simulink model "PS3"  (Simulink 7.3)
settings: Solver=ode5  StartTime=0.0  StopTime=inf  FixedStep=0.1  RelTol=1e-3
libraries: simulink x18, dspinverses x1
settings Model: Creator=Dinh  LastModifiedBy=mcl  BufferReuse=off
settings DataIOCC: LimitDataPoints=off  SaveOutput=off  SaveTime=off
settings OptimizationCC: BlockReduction=off  BooleanDataType=off  ConditionallyExecuteInputs=off  OptimizeBlockIOStorage=off  BufferReuse=off  ExpressionFolding=off  LocalBlockOutputs=off  SimCompilerOptimization=On
settings SFSimCC: SimBuildMode=sf_nonincremental_build
settings RTWCC: SystemTargetFile=nidll.tlc  TemplateMakefile=nidll_vc.tmf  Description=NI Real-Time Target for Release 2007b or later  ProcessScript=nidll_make_rtw_hook
settings STFCustomTargetCC: MatFileLogging=on  SystemTargetFile=nidll.tlc

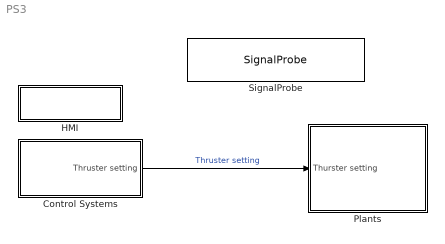
== system PS3 ==
  Control Systems : Subsystem
  HMI : Subsystem
  Plants : Subsystem
  SignalProbe : S-Function  Description=Use this block with SIT.  FunctionName=SignalProbe  Parameters=1  EnableBusSupport=off
      settings: PreSaveFcn=NISIT_ModelVars;
      mask Description: The LabVIEW Simulation Interface Toolkit uses the SignalProbe block to probe the signals in the model. The SignalProbe block must be on the top level of the model hierarchy. You can have only one SignalProbe block per model file. Do not rename the SignalProbe block. Do not change the name of another model block to SignalProbe.
  wires:
  Control Systems/1(Thruster setting) -> Plants/1(Thurster setting)  "Thruster setting"

== system PS3/Control Systems ==
  note: 0 - PS3 u input control
      | 1 - PS3 tau input control
  Control Mode : Constant  Value=0
  PS3 input : Subsystem
  PS3 tau input control : Subsystem
      settings: MinAlgLoopOccurrences=on
  PS3 u input control : Subsystem
      settings: MinAlgLoopOccurrences=on
  Saturation : Saturate  UpperLimit=1.0  LowerLimit=-1.0
  Thruster setting Switch : MultiPortSwitch  Inputs=2  zeroidx=on
  Thruster setting : Outport  PortDimensions=7
  wires:
  Thruster setting Switch/1 -> Saturation/1
  Saturation/1 -> Thruster setting/1
  PS3 input/1(DuelShock 3 signals) -> PS3 u input control/1(PS3 Signals), PS3 tau input control/1(PS3 Signals)
  PS3 input/2(PS3 BT Power) -> PS3 u input control/2(PS3 BT Power), PS3 tau input control/2(PS3 BT Power)
  PS3 input/3(PS3 VSP Speed) -> PS3 u input control/3(PS3 VSP Speed), PS3 tau input control/3(PS3 VSP Speed)
  Control Mode/1 -> Thruster setting Switch/1
  PS3 u input control/1(Thruster setting) -> Thruster setting Switch/2
  PS3 tau input control/1(Thruster setting) -> Thruster setting Switch/3

== system PS3/HMI ==
  Battery Bow Thruster : Gain  ParameterDataType=fixdt(1, 16)  ParameterScaling=2^0  OutDataType=fixdt(1, 16)  OutScaling=2^0
  Battery Main : Gain  Gain=2  ParameterDataType=fixdt(1, 16)  ParameterScaling=2^0  OutDataType=fixdt(1, 16)  OutScaling=2^0
  Battery Servo : Gain  ParameterDataType=fixdt(1, 16)  ParameterScaling=2^0  OutDataType=fixdt(1, 16)  OutScaling=2^0
  SIT zAI0 : S-Function  Priority=1  FunctionName=NI_SIT_IO  Parameters=width dtype portnum stime stype btype  EnableBusSupport=off  mask(SIT Inport){portnum=1, width=-1, stime=-1, dtype=auto, stype=auto, btype=1}
      mask prompts: portnum "Port number:"; width "Port dimensions (-1 for dynamically sized):"; stime "Sample time (-1 for inherited):"; dtype "Data type:"; stype "Signal type:"; btype "Block type:"
      mask help: Use this inport on any level of nested subsystems to allow the LabVIEW Simulation Interface Toolkit to map hardware to it.
      mask init:
      | NI_SIT_IO_init;
      settings: CopyFcn=NI_SIT_IO_callbacks(1);  DeleteFcn=NI_SIT_IO_callbacks(2);
      mask StyleString: edit,edit,edit,popup(auto|double|single|int8|uint8|int16|uint16|int32|uint32|boolean),popup(auto|real|complex),edit
      mask CallbackString: NI_SIT_IO_callbacks(3);|||NI_SIT_IO_callbacks(4);||
      mask TabNameString: Parameters,Parameters,Parameters,Parameters,Parameters,Parameters
      mask Display:
      | patch([-x x], [-y y], [.90980 .81960 .32156]);
      | plot([0 -x x 0], [rad -y y rad]);
      | fprintf('SIT%d', portnum);
  SIT zAI1 : S-Function  Priority=2  FunctionName=NI_SIT_IO  Parameters=width dtype portnum stime stype btype  EnableBusSupport=off  mask(SIT Inport){portnum=2, width=-1, stime=-1, dtype=auto, stype=auto, btype=1}
      mask prompts: portnum "Port number:"; width "Port dimensions (-1 for dynamically sized):"; stime "Sample time (-1 for inherited):"; dtype "Data type:"; stype "Signal type:"; btype "Block type:"
      mask help: Use this inport on any level of nested subsystems to allow the LabVIEW Simulation Interface Toolkit to map hardware to it.
      mask init:
      | NI_SIT_IO_init;
      settings: CopyFcn=NI_SIT_IO_callbacks(1);  DeleteFcn=NI_SIT_IO_callbacks(2);
      mask StyleString: edit,edit,edit,popup(auto|double|single|int8|uint8|int16|uint16|int32|uint32|boolean),popup(auto|real|complex),edit
      mask CallbackString: NI_SIT_IO_callbacks(3);|||NI_SIT_IO_callbacks(4);||
      mask TabNameString: Parameters,Parameters,Parameters,Parameters,Parameters,Parameters
      mask Display:
      | patch([-x x], [-y y], [.90980 .81960 .32156]);
      | plot([0 -x x 0], [rad -y y rad]);
      | fprintf('SIT%d', portnum);
  SIT zAI2 : S-Function  Priority=3  FunctionName=NI_SIT_IO  Parameters=width dtype portnum stime stype btype  EnableBusSupport=off  mask(SIT Inport){portnum=3, width=-1, stime=-1, dtype=auto, stype=auto, btype=1}
      mask prompts: portnum "Port number:"; width "Port dimensions (-1 for dynamically sized):"; stime "Sample time (-1 for inherited):"; dtype "Data type:"; stype "Signal type:"; btype "Block type:"
      mask help: Use this inport on any level of nested subsystems to allow the LabVIEW Simulation Interface Toolkit to map hardware to it.
      mask init:
      | NI_SIT_IO_init;
      settings: CopyFcn=NI_SIT_IO_callbacks(1);  DeleteFcn=NI_SIT_IO_callbacks(2);
      mask StyleString: edit,edit,edit,popup(auto|double|single|int8|uint8|int16|uint16|int32|uint32|boolean),popup(auto|real|complex),edit
      mask CallbackString: NI_SIT_IO_callbacks(3);|||NI_SIT_IO_callbacks(4);||
      mask TabNameString: Parameters,Parameters,Parameters,Parameters,Parameters,Parameters
      mask Display:
      | patch([-x x], [-y y], [.90980 .81960 .32156]);
      | plot([0 -x x 0], [rad -y y rad]);
      | fprintf('SIT%d', portnum);
  Terminator Bow Thruster Battery : Terminator
  Terminator Main Battery : Terminator
  Terminator Servo Battery : Terminator
  wires:
  SIT zAI0/1 -> Battery Bow Thruster/1
  SIT zAI1/1 -> Battery Servo/1
  SIT zAI2/1 -> Battery Main/1
  Battery Bow Thruster/1 -> Terminator Bow Thruster Battery/1
  Battery Servo/1 -> Terminator Servo Battery/1
  Battery Main/1 -> Terminator Main Battery/1

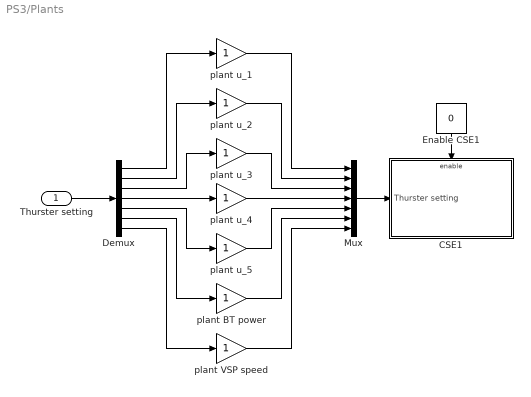
== system PS3/Plants ==
  Thurster setting : Inport
  CSE1 : Subsystem
  Demux : Demux  Outputs=7
  Enable CSE1 : Constant  Value=0
  Mux : Mux  Inputs=7
  plant BT power : Gain  ParameterDataType=fixdt(1, 16)  ParameterScaling=2^0  OutDataType=fixdt(1, 16)  OutScaling=2^0
  plant VSP speed : Gain  ParameterDataType=fixdt(1, 16)  ParameterScaling=2^0  OutDataType=fixdt(1, 16)  OutScaling=2^0
  plant u_{1..5} (5 alike) : Gain  ParameterDataType=fixdt(1, 16)  ParameterScaling=2^0  OutDataType=fixdt(1, 16)  OutScaling=2^0
  wires:
  Enable CSE1/1 -> CSE1/Enable
  Thurster setting/1 -> Demux/1
  Mux/1 -> CSE1/1(Thurster setting)
  Demux/1 -> plant u_1/1
  Demux/2 -> plant u_2/1
  Demux/3 -> plant u_3/1
  Demux/4 -> plant u_4/1
  plant u_4/1 -> Mux/4
  plant u_1/1 -> Mux/1
  plant u_2/1 -> Mux/2
  plant u_3/1 -> Mux/3
  Demux/5 -> plant u_5/1
  Demux/6 -> plant BT power/1
  Demux/7 -> plant VSP speed/1
  plant u_5/1 -> Mux/5
  plant BT power/1 -> Mux/6
  plant VSP speed/1 -> Mux/7

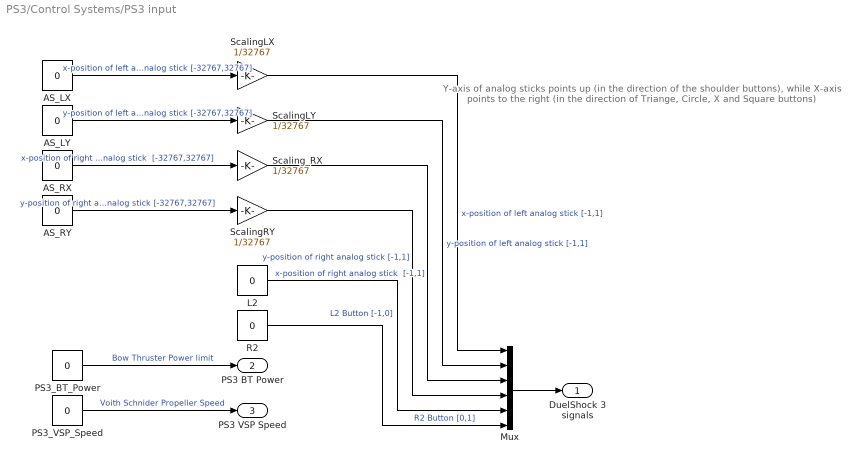
== system PS3/Control Systems/PS3 input ==
  note: Y-axis of analog sticks points up (in the direction of the shoulder buttons),
      | while  X-axis points to the right (in the direction of
      | Triange, Circle, X and Square buttons)
  AS_LX : Constant  Value=0
  AS_LY : Constant  Value=0
  AS_RX : Constant  Value=0
  AS_RY : Constant  Value=0
  L2 : Constant  Value=0
  Mux : Mux  Inputs=6
  PS3_BT_Power : Constant  Value=0
  PS3_VSP_Speed : Constant  Value=0
  R2 : Constant  Value=0
  ScalingLX : Gain  Gain=1/32767
  ScalingLY : Gain  Gain=1/32767
  ScalingRY : Gain  Gain=1/32767
  Scaling_RX : Gain  Gain=1/32767
  DuelShock 3 signals : Outport
  PS3 BT Power : Outport  Port=2
  PS3 VSP Speed : Outport  Port=3
  wires:
  PS3_VSP_Speed/1 -> PS3 VSP Speed/1  "Voith Schnider Propeller Speed"
  PS3_BT_Power/1 -> PS3 BT Power/1  "Bow Thruster Power limit"
  Mux/1 -> DuelShock 3 signals/1
  AS_LX/1 -> ScalingLX/1  "x-position of left analog stick [-32767,32767]"
  ScalingLX/1 -> Mux/1  "x-position of left analog stick [-1,1]"
  AS_LY/1 -> ScalingLY/1  "y-position of left analog stick [-32767,32767]"
  ScalingLY/1 -> Mux/2  "y-position of left analog stick [-1,1]"
  AS_RX/1 -> Scaling_RX/1  "x-position of right analog stick  [-32767,32767]"
  Scaling_RX/1 -> Mux/3  "x-position of right analog stick  [-1,1]"
  ScalingRY/1 -> Mux/4  "y-position of right analog stick [-1,1]"
  AS_RY/1 -> ScalingRY/1  "y-position of right analog stick [-32767,32767]"
  L2/1 -> Mux/5  "L2 Button [-1,0]"
  R2/1 -> Mux/6  "R2 Button [0,1]"

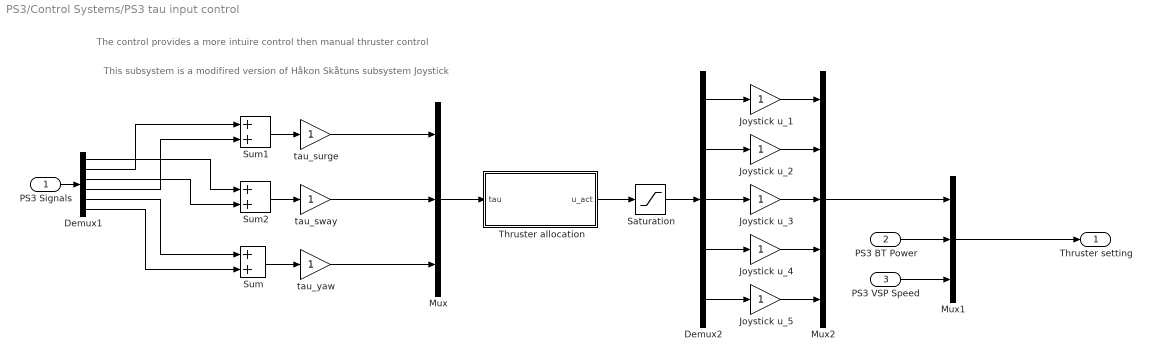
== system PS3/Control Systems/PS3 tau input control ==
  note: The control provides a more intuire control then manual thruster control
  note: This subsystem is a modifired version of Håkon Skåtuns subsystem Joystick
  PS3 Signals : Inport
  PS3 BT Power : Inport  Port=2
  PS3 VSP Speed : Inport  Port=3
  Demux1 : Demux  Outputs=6
  Demux2 : Demux  Outputs=5
  Joystick u_{1..5} (5 alike) : Gain  ParameterDataType=fixdt(1, 16)  ParameterScaling=2^0  OutDataType=fixdt(1, 16)  OutScaling=2^0
  Mux : Mux  Inputs=3
  Mux1 : Mux  Inputs=3
  Mux2 : Mux  Inputs=5
  Saturation : Saturate  UpperLimit=1.0  LowerLimit=-1.0
  Sum : Sum
  Sum1 : Sum
  Sum2 : Sum
  Thruster allocation : Subsystem
  tau_surge : Gain
  tau_sway : Gain
  tau_yaw : Gain
  Thruster setting : Outport
  wires:
  PS3 Signals/1 -> Demux1/1
  Demux1/5 -> Sum/1
  Demux1/6 -> Sum/2
  Sum/1 -> tau_yaw/1
  Mux/1 -> Thruster allocation/1(tau)
  Mux1/1 -> Thruster setting/1
  PS3 BT Power/1 -> Mux1/2
  PS3 VSP Speed/1 -> Mux1/3
  Thruster allocation/1(u_act) -> Saturation/1
  Demux1/4 -> Sum1/2
  Demux1/2 -> Sum1/1
  Sum1/1 -> tau_surge/1
  Demux1/1 -> Sum2/1
  Demux1/3 -> Sum2/2
  Sum2/1 -> tau_sway/1
  Demux2/1 -> Joystick u_1/1
  Demux2/2 -> Joystick u_2/1
  Demux2/3 -> Joystick u_3/1
  Joystick u_1/1 -> Mux2/1
  Joystick u_3/1 -> Mux2/3
  Joystick u_2/1 -> Mux2/2
  Demux2/4 -> Joystick u_4/1
  Demux2/5 -> Joystick u_5/1
  Joystick u_4/1 -> Mux2/4
  Joystick u_5/1 -> Mux2/5
  Saturation/1 -> Demux2/1
  Mux2/1 -> Mux1/1
  tau_surge/1 -> Mux/1
  tau_sway/1 -> Mux/2
  tau_yaw/1 -> Mux/3

== system PS3/Control Systems/PS3 u input control ==
  note: Manuel thruster control is intended for testing and flexing of thrusters and its signals
  note: Mapping PS3 signals to thruster settings:
      | - Y-position controls surge force of VSP
      | - X-positon controls sway force of VSP
      | - Left Analogstick controls port VSP
      | - Right Analogstick controls starboard VSP
      | - Postive values gives postive motions and vice versa
      | - R2 pressed gives postive yaw motion
      | - L2 pressed gives negative yaw motion
  note: This subsystem is a modifired version of Håkon Skåtuns subsystem Manual Control
  PS3 Signals : Inport
  PS3 BT Power : Inport  Port=2
  PS3 VSP Speed : Inport  Port=3
  Add : Sum  Inputs=|++
  Demux : Demux  Outputs=6
  Mux : Mux  Inputs=7
  PS3 u_{1..5} (5 alike) : Gain  ParameterDataType=fixdt(1, 16)  ParameterScaling=2^0  OutDataType=fixdt(1, 16)  OutScaling=2^0
  Thruster setting : Outport
  wires:
  PS3 Signals/1 -> Demux/1
  Demux/1 -> PS3 u_2/1  "Left/Right position of Left Analogstick"
  Demux/2 -> PS3 u_1/1  "Up/Down position of Left Analogstick"
  Demux/3 -> PS3 u_4/1  "Left/Right position of Right Analogstick"
  Demux/4 -> PS3 u_3/1  "Up/Down position of Right Analogstick"
  Demux/5 -> Add/1  "L2 signal"
  Demux/6 -> Add/2  "R2 signal"
  PS3 VSP Speed/1 -> Mux/7  "VPS Speed"
  PS3 BT Power/1 -> Mux/6  "Bow Thruster Limit"
  Add/1 -> PS3 u_5/1  "Bow Thruster direction"
  Mux/1 -> Thruster setting/1
  PS3 u_1/1 -> Mux/1  "u_1"
  PS3 u_2/1 -> Mux/2  "u_2"
  PS3 u_5/1 -> Mux/5  "u_5"
  PS3 u_4/1 -> Mux/4  "u_4"
  PS3 u_3/1 -> Mux/3  "u_3"

== system PS3/Plants/CSE1 ==
  note: This subsystem is a modifired version of Håkon Skåtuns subsystem CSE1
  Thurster setting : Inport
  Enable : EnablePort  StatesWhenEnabling=reset
  Bow Thruster : Subsystem
  Demux : Demux  Outputs=7
  "Voith Schneider Propeller " : Subsystem
  wires:
  Thurster setting/1 -> Demux/1
  Demux/1 -> "Voith Schneider Propeller "/1(Port VSP y u_1)
  Demux/2 -> "Voith Schneider Propeller "/2(Port VSP x u_2)
  Demux/3 -> "Voith Schneider Propeller "/3(Starboard VSP y u_3)
  Demux/4 -> "Voith Schneider Propeller "/4(Starboard VSP x u_4)
  Demux/7 -> "Voith Schneider Propeller "/5(VSP Speed)
  Demux/5 -> Bow Thruster/1(Bow Thruster Direction u_5)
  Demux/6 -> Bow Thruster/2(Bow Thruster Power)

== system PS3/Control Systems/PS3 tau input control/Thruster allocation ==
  tau : Inport
  f_act to u_act : Subsystem
  tau to f_act : Subsystem
  u_act : Outport
  wires:
  tau/1 -> tau to f_act/1(tau)
  tau to f_act/1(f_act) -> f_act to u_act/1(f_act)
  f_act to u_act/1(u_act) -> u_act/1

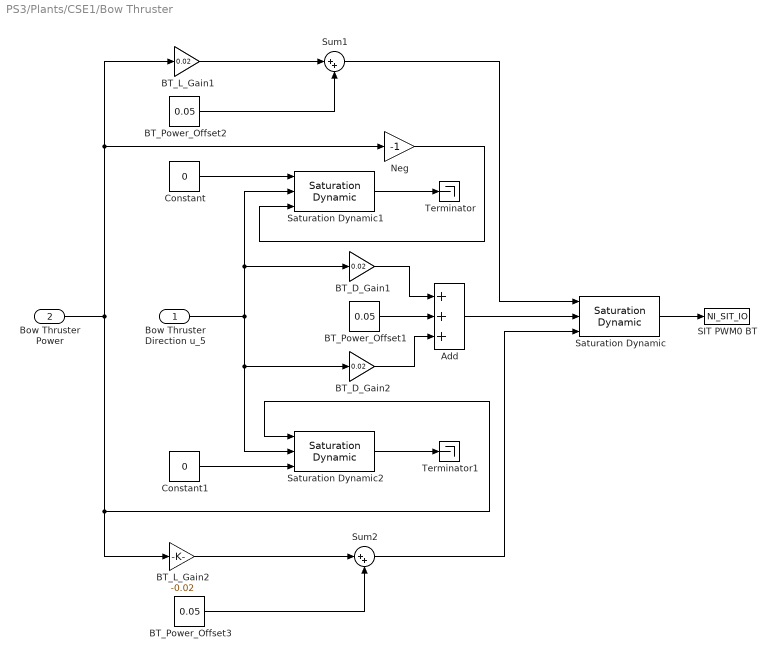
== system PS3/Plants/CSE1/Bow Thruster ==
  Bow Thruster Direction u_5 : Inport
  Bow Thruster Power : Inport  Port=2
  Add : Sum  Inputs=+++
  BT_D_Gain1 : Gain  Gain=0.02
  BT_D_Gain2 : Gain  Gain=0.02
  BT_L_Gain1 : Gain  Gain=0.02
  BT_L_Gain2 : Gain  Gain=-0.02
  BT_Power_Offset1 : Constant  Value=0.05
  BT_Power_Offset2 : Constant  Value=0.05
  BT_Power_Offset3 : Constant  Value=0.05
  Constant : Constant  Value=0  OutDataType=fixdt(1, 16)  OutScaling=2^0
  Constant1 : Constant  Value=0  OutDataType=fixdt(1, 16)  OutScaling=2^0
  Neg : Gain  Gain=-1  ParameterDataType=fixdt(1, 16)  ParameterScaling=2^0  OutDataType=fixdt(1, 16)  OutScaling=2^0
  SIT PWM0 BT : S-Function  Priority=1  FunctionName=NI_SIT_IO  Parameters=width dtype portnum stime stype btype  EnableBusSupport=off  mask(SIT Outport){portnum=1, width=-1, stime=-1, dtype=auto, stype=auto, btype=0}
      mask prompts: portnum "Port number:"; width "Port dimensions (-1 for dynamically sized):"; stime "Sample time (-1 for inherited):"; dtype "Data type:"; stype "Signal type:"; btype "Block type:"
      mask help: Use this outport on any level of nested subsystems to allow the LabVIEW Simulation Interface Toolkit to map hardware to it.
      mask init:
      | NI_SIT_IO_init;
      settings: CopyFcn=NI_SIT_IO_callbacks(1);  DeleteFcn=NI_SIT_IO_callbacks(2);
      mask StyleString: edit,edit,edit,popup(auto|double|single|int8|uint8|int16|uint16|int32|uint32|boolean),popup(auto|real|complex),edit
      mask CallbackString: NI_SIT_IO_callbacks(3);|||NI_SIT_IO_callbacks(4);||
      mask TabNameString: Parameters,Parameters,Parameters,Parameters,Parameters,Parameters
      mask Display:
      | patch([-x x], [-y y], [.90980 .81960 .32156]);
      | plot([0 -x x 0], [rad -y y rad]);
      | fprintf('SIT%d', portnum);
  Saturation Dynamic : simulink/Discontinuities/Saturation Dynamic  SystemSampleTime=-1  OutMin=[]  OutMax=[]  OutDataTypeStr=Inherit: Same as second input  OutDataType=fixdt(1, 16)  OutScaling=2^-10  DoSatur=off
  Saturation Dynamic1 : simulink/Discontinuities/Saturation Dynamic  SystemSampleTime=-1  OutMin=[]  OutMax=[]  OutDataTypeStr=Inherit: Same as second input  OutDataType=fixdt(1, 16)  OutScaling=2^-10  DoSatur=off
  Saturation Dynamic2 : simulink/Discontinuities/Saturation Dynamic  SystemSampleTime=-1  OutMin=[]  OutMax=[]  OutDataTypeStr=Inherit: Same as second input  OutDataType=fixdt(1, 16)  OutScaling=2^-10  DoSatur=off
  Sum1 : Sum  Inputs=|++
  Sum2 : Sum  Inputs=|++
  Terminator : Terminator
  Terminator1 : Terminator
  wires:
  Bow Thruster Direction u_5/1 -> BT_D_Gain1/1, Saturation Dynamic1/2, BT_D_Gain2/1, Saturation Dynamic2/2
  BT_D_Gain1/1 -> Add/1
  BT_D_Gain2/1 -> Add/3
  BT_Power_Offset1/1 -> Add/2
  Add/1 -> Saturation Dynamic/2
  Bow Thruster Power/1 -> BT_L_Gain2/1, Saturation Dynamic2/1, BT_L_Gain1/1, Neg/1
  Sum1/1 -> Saturation Dynamic/1
  BT_L_Gain1/1 -> Sum1/1
  BT_L_Gain2/1 -> Sum2/1
  Sum2/1 -> Saturation Dynamic/3
  BT_Power_Offset2/1 -> Sum1/2
  BT_Power_Offset3/1 -> Sum2/2
  Saturation Dynamic/1 -> SIT PWM0 BT/1
  Saturation Dynamic2/1 -> Terminator1/1
  Saturation Dynamic1/1 -> Terminator/1
  Constant/1 -> Saturation Dynamic1/1
  Constant1/1 -> Saturation Dynamic2/3
  Neg/1 -> Saturation Dynamic1/3

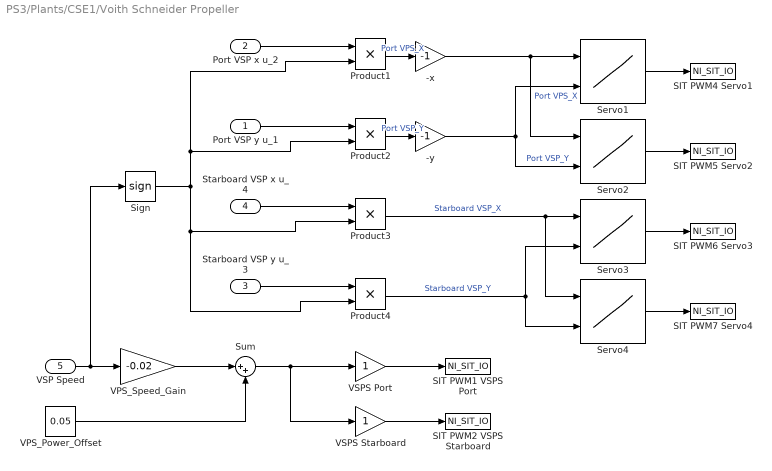
== system PS3/Plants/CSE1/Voith Schneider Propeller  ==
  Port VSP y u_1 : Inport
  Port VSP x u_2 : Inport  Port=2
  Starboard VSP y u_3 : Inport  Port=3
  Starboard VSP x u_4 : Inport  Port=4
  VSP Speed : Inport  Port=5
  -x : Gain  Gain=-1
  -y : Gain  Gain=-1
  Product{1..4} (4 alike) : Product  RndMeth=Zero
  SIT PWM1 VSPS Port : S-Function  Priority=5  FunctionName=NI_SIT_IO  Parameters=width dtype portnum stime stype btype  EnableBusSupport=off  mask(SIT Outport){portnum=5, width=-1, stime=-1, dtype=auto, stype=auto, btype=0}
      mask prompts: portnum "Port number:"; width "Port dimensions (-1 for dynamically sized):"; stime "Sample time (-1 for inherited):"; dtype "Data type:"; stype "Signal type:"; btype "Block type:"
      mask help: Use this outport on any level of nested subsystems to allow the LabVIEW Simulation Interface Toolkit to map hardware to it.
      mask init:
      | NI_SIT_IO_init;
      settings: CopyFcn=NI_SIT_IO_callbacks(1);  DeleteFcn=NI_SIT_IO_callbacks(2);
      mask StyleString: edit,edit,edit,popup(auto|double|single|int8|uint8|int16|uint16|int32|uint32|boolean),popup(auto|real|complex),edit
      mask CallbackString: NI_SIT_IO_callbacks(3);|||NI_SIT_IO_callbacks(4);||
      mask TabNameString: Parameters,Parameters,Parameters,Parameters,Parameters,Parameters
      mask Display:
      | patch([-x x], [-y y], [.90980 .81960 .32156]);
      | plot([0 -x x 0], [rad -y y rad]);
      | fprintf('SIT%d', portnum);
  SIT PWM2 VSPS Starboard : S-Function  Priority=6  FunctionName=NI_SIT_IO  Parameters=width dtype portnum stime stype btype  EnableBusSupport=off  mask(SIT Outport){portnum=6, width=-1, stime=-1, dtype=auto, stype=auto, btype=0}
      mask prompts: portnum "Port number:"; width "Port dimensions (-1 for dynamically sized):"; stime "Sample time (-1 for inherited):"; dtype "Data type:"; stype "Signal type:"; btype "Block type:"
      mask help: Use this outport on any level of nested subsystems to allow the LabVIEW Simulation Interface Toolkit to map hardware to it.
      mask init:
      | NI_SIT_IO_init;
      settings: CopyFcn=NI_SIT_IO_callbacks(1);  DeleteFcn=NI_SIT_IO_callbacks(2);
      mask StyleString: edit,edit,edit,popup(auto|double|single|int8|uint8|int16|uint16|int32|uint32|boolean),popup(auto|real|complex),edit
      mask CallbackString: NI_SIT_IO_callbacks(3);|||NI_SIT_IO_callbacks(4);||
      mask TabNameString: Parameters,Parameters,Parameters,Parameters,Parameters,Parameters
      mask Display:
      | patch([-x x], [-y y], [.90980 .81960 .32156]);
      | plot([0 -x x 0], [rad -y y rad]);
      | fprintf('SIT%d', portnum);
  SIT PWM4 Servo1 : S-Function  Priority=1  FunctionName=NI_SIT_IO  Parameters=width dtype portnum stime stype btype  EnableBusSupport=off  mask(SIT Outport){portnum=1, width=-1, stime=-1, dtype=auto, stype=auto, btype=0}
      mask prompts: portnum "Port number:"; width "Port dimensions (-1 for dynamically sized):"; stime "Sample time (-1 for inherited):"; dtype "Data type:"; stype "Signal type:"; btype "Block type:"
      mask help: Use this outport on any level of nested subsystems to allow the LabVIEW Simulation Interface Toolkit to map hardware to it.
      mask init:
      | NI_SIT_IO_init;
      settings: CopyFcn=NI_SIT_IO_callbacks(1);  DeleteFcn=NI_SIT_IO_callbacks(2);
      mask StyleString: edit,edit,edit,popup(auto|double|single|int8|uint8|int16|uint16|int32|uint32|boolean),popup(auto|real|complex),edit
      mask CallbackString: NI_SIT_IO_callbacks(3);|||NI_SIT_IO_callbacks(4);||
      mask TabNameString: Parameters,Parameters,Parameters,Parameters,Parameters,Parameters
      mask Display:
      | patch([-x x], [-y y], [.90980 .81960 .32156]);
      | plot([0 -x x 0], [rad -y y rad]);
      | fprintf('SIT%d', portnum);
  SIT PWM5 Servo2 : S-Function  Priority=2  FunctionName=NI_SIT_IO  Parameters=width dtype portnum stime stype btype  EnableBusSupport=off  mask(SIT Outport){portnum=2, width=-1, stime=-1, dtype=auto, stype=auto, btype=0}
      mask prompts: portnum "Port number:"; width "Port dimensions (-1 for dynamically sized):"; stime "Sample time (-1 for inherited):"; dtype "Data type:"; stype "Signal type:"; btype "Block type:"
      mask help: Use this outport on any level of nested subsystems to allow the LabVIEW Simulation Interface Toolkit to map hardware to it.
      mask init:
      | NI_SIT_IO_init;
      settings: CopyFcn=NI_SIT_IO_callbacks(1);  DeleteFcn=NI_SIT_IO_callbacks(2);
      mask StyleString: edit,edit,edit,popup(auto|double|single|int8|uint8|int16|uint16|int32|uint32|boolean),popup(auto|real|complex),edit
      mask CallbackString: NI_SIT_IO_callbacks(3);|||NI_SIT_IO_callbacks(4);||
      mask TabNameString: Parameters,Parameters,Parameters,Parameters,Parameters,Parameters
      mask Display:
      | patch([-x x], [-y y], [.90980 .81960 .32156]);
      | plot([0 -x x 0], [rad -y y rad]);
      | fprintf('SIT%d', portnum);
  SIT PWM6 Servo3 : S-Function  Priority=3  FunctionName=NI_SIT_IO  Parameters=width dtype portnum stime stype btype  EnableBusSupport=off  mask(SIT Outport){portnum=3, width=-1, stime=-1, dtype=auto, stype=auto, btype=0}
      mask prompts: portnum "Port number:"; width "Port dimensions (-1 for dynamically sized):"; stime "Sample time (-1 for inherited):"; dtype "Data type:"; stype "Signal type:"; btype "Block type:"
      mask help: Use this outport on any level of nested subsystems to allow the LabVIEW Simulation Interface Toolkit to map hardware to it.
      mask init:
      | NI_SIT_IO_init;
      settings: CopyFcn=NI_SIT_IO_callbacks(1);  DeleteFcn=NI_SIT_IO_callbacks(2);
      mask StyleString: edit,edit,edit,popup(auto|double|single|int8|uint8|int16|uint16|int32|uint32|boolean),popup(auto|real|complex),edit
      mask CallbackString: NI_SIT_IO_callbacks(3);|||NI_SIT_IO_callbacks(4);||
      mask TabNameString: Parameters,Parameters,Parameters,Parameters,Parameters,Parameters
      mask Display:
      | patch([-x x], [-y y], [.90980 .81960 .32156]);
      | plot([0 -x x 0], [rad -y y rad]);
      | fprintf('SIT%d', portnum);
  SIT PWM7 Servo4 : S-Function  Priority=4  FunctionName=NI_SIT_IO  Parameters=width dtype portnum stime stype btype  EnableBusSupport=off  mask(SIT Outport){portnum=4, width=-1, stime=-1, dtype=auto, stype=auto, btype=0}
      mask prompts: portnum "Port number:"; width "Port dimensions (-1 for dynamically sized):"; stime "Sample time (-1 for inherited):"; dtype "Data type:"; stype "Signal type:"; btype "Block type:"
      mask help: Use this outport on any level of nested subsystems to allow the LabVIEW Simulation Interface Toolkit to map hardware to it.
      mask init:
      | NI_SIT_IO_init;
      settings: CopyFcn=NI_SIT_IO_callbacks(1);  DeleteFcn=NI_SIT_IO_callbacks(2);
      mask StyleString: edit,edit,edit,popup(auto|double|single|int8|uint8|int16|uint16|int32|uint32|boolean),popup(auto|real|complex),edit
      mask CallbackString: NI_SIT_IO_callbacks(3);|||NI_SIT_IO_callbacks(4);||
      mask TabNameString: Parameters,Parameters,Parameters,Parameters,Parameters,Parameters
      mask Display:
      | patch([-x x], [-y y], [.90980 .81960 .32156]);
      | plot([0 -x x 0], [rad -y y rad]);
      | fprintf('SIT%d', portnum);
  Servo1 : Lookup2D  RowIndex=[-1,0,1]  ColumnIndex=[-1,0,1]  Table=reshape([0.06,0.0495363,0.043301,0.06,0.052446,0.043301,0.06,0.0541518,0.043301],3,3)
  Servo2 : Lookup2D  RowIndex=[-1,0,1]  ColumnIndex=[-1,0,1]  Table=reshape([0.03860880,0.0386088,0.03860880,0.0459941,0.0477243,0.0500953,0.057,0.057,0.057],3,3)
  Servo3 : Lookup2D  RowIndex=[-1,0,1]  ColumnIndex=[-1,0,1]  Table=reshape([0.0640809,0.0640809,0.0640809,0.0539629,0.0541315,0.0556492,0.0442664,0.0442664,0.0442664],3,3)
  Servo4 : Lookup2D  RowIndex=[-1,0,1]  ColumnIndex=[-1,0,1]  Table=reshape([0.0602867,0.0470489,0.0403879,0.0602867,0.049747,0.0403879,0.0602867,0.0526138,0.0403879],3,3)
  Sign : Signum
  Sum : Sum  Inputs=|++
  VPS_Power_Offset : Constant  Value=0.05
  VPS_Speed_Gain : Gain  Gain=-0.02
  VSPS Port : Gain  ParameterDataType=fixdt(1, 16)  ParameterScaling=2^0  OutDataType=fixdt(1, 16)  OutScaling=2^0
  VSPS Starboard : Gain  ParameterDataType=fixdt(1, 16)  ParameterScaling=2^0  OutDataType=fixdt(1, 16)  OutScaling=2^0
  wires:
  Sign/1 -> Product1/2, Product2/2, Product3/2, Product4/2
  Product1/1 -> -x/1  "Port VPS_X"
  Product2/1 -> -y/1  "Port VSP_Y"
  Servo1/1 -> SIT PWM4 Servo1/1
  Servo2/1 -> SIT PWM5 Servo2/1
  Product3/1 -> Servo3/1, Servo4/1  "Starboard VSP_X"
  Product4/1 -> Servo3/2, Servo4/2  "Starboard VSP_Y"
  Servo3/1 -> SIT PWM6 Servo3/1
  Servo4/1 -> SIT PWM7 Servo4/1
  VSP Speed/1 -> VPS_Speed_Gain/1, Sign/1
  VPS_Speed_Gain/1 -> Sum/1
  VPS_Power_Offset/1 -> Sum/2
  Sum/1 -> VSPS Port/1, VSPS Starboard/1
  -y/1 -> Servo2/2, Servo1/2  "Port VSP_Y"
  -x/1 -> Servo1/1, Servo2/1  "Port VPS_X"
  Starboard VSP y u_3/1 -> Product4/1
  Starboard VSP x u_4/1 -> Product3/1
  Port VSP y u_1/1 -> Product2/1
  Port VSP x u_2/1 -> Product1/1
  VSPS Port/1 -> SIT PWM1 VSPS Port/1
  VSPS Starboard/1 -> SIT PWM2 VSPS Starboard/1

== system PS3/Control Systems/PS3 tau input control/Thruster allocation/f_act to u_act ==
  f_act : Inport
  Demux : Demux  Outputs=5
  Mux : Mux  Inputs=5
  f_1 to u_1 : Subsystem
  f_2 to u_2 : Subsystem
  f_3 to u_3 : Subsystem
  f_4 to u_4 : Subsystem
  f_5 to u_5 : Subsystem
  u_act : Outport
  wires:
  f_5 to u_5/1(u_5) -> Mux/5
  f_4 to u_4/1(u_4) -> Mux/4
  f_3 to u_3/1(u_3) -> Mux/3
  f_2 to u_2/1(u_2) -> Mux/2
  f_1 to u_1/1(u_1) -> Mux/1
  Demux/5 -> f_5 to u_5/1(f_5)
  Demux/4 -> f_4 to u_4/1(f_4)
  Demux/3 -> f_3 to u_3/1(f_3)
  Demux/1 -> f_1 to u_1/1(f_1)
  Mux/1 -> u_act/1
  f_act/1 -> Demux/1
  Demux/2 -> f_2 to u_2/1(f_2)

== system PS3/Control Systems/PS3 tau input control/Thruster allocation/tau to f_act ==
  tau : Inport
  Product : Product  Multiplication=Matrix(*)  OutDataType=fixdt(1, 16)  OutScaling=2^0  RndMeth=Zero
  Pseudoinverse : dspinverses/Pseudoinverse  wanterr=off
  T_e : Subsystem
  f_act : Outport
  wires:
  Product/1 -> f_act/1
  tau/1 -> Product/2
  Pseudoinverse/1 -> Product/1
  T_e/1(T_e) -> Pseudoinverse/1

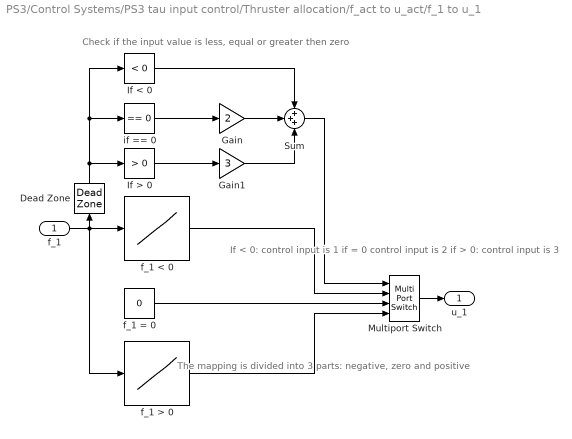
== system PS3/Control Systems/PS3 tau input control/Thruster allocation/f_act to u_act/f_1 to u_1 ==
  note: If < 0: control input is 1
      | if = 0 control input is 2
      | if > 0: control input is 3
  note: Check if the input value is less, equal or greater then zero
  note: The mapping is divided into 3 parts:
      | negative, zero and positive
  f_1 : Inport
  Dead Zone : DeadZone  LowerValue=-0.001  UpperValue=0.001  SaturateOnIntegerOverflow=on
  Gain : Gain  Gain=2  ParameterDataType=fixdt(1, 16)  ParameterScaling=2^0  OutDataType=fixdt(1, 16)  OutScaling=2^0
  Gain1 : Gain  Gain=3  ParameterDataType=fixdt(1, 16)  ParameterScaling=2^0  OutDataType=fixdt(1, 16)  OutScaling=2^0
  If < 0 : simulink/Logic and Bit Operations/Compare To Constant  SystemSampleTime=-1  relop=<  const=0  LogicOutDataTypeMode=uint8
  If > 0 : simulink/Logic and Bit Operations/Compare To Constant  SystemSampleTime=-1  relop=>  const=0  LogicOutDataTypeMode=uint8
  Multiport Switch : MultiPortSwitch  OutDataType=fixdt(1, 16)  OutScaling=2^0
  Sum : Sum  Inputs=+++  OutDataType=fixdt(1, 16)  OutScaling=2^0
  f_1 < 0 : Lookup  InputValues=|  Table=|  LookUpMeth=Interpolation-Use End Values  OutDataType=fixdt(1, 16)  OutScaling=2^0
      InputValues=|
      | [-1.324
      | -1.169
      | -0.919
      | -0.703
      | -0.535
      | -0.292
      | -0.165
      | -0.060
      | 0]
      Table=|
      | [-1.0000
      |    -0.9000
      |    -0.8000
      |    -0.7000
      |    -0.6000
      |    -0.5000
      |    -0.4000
      |    -0.3000
      |    -0.2089]
  f_1 = 0 : Constant  Value=0  OutDataType=fixdt(1, 16)  OutScaling=2^0
  f_1 > 0 : Lookup  InputValues=|  Table=|  LookUpMeth=Interpolation-Use End Values  OutDataType=fixdt(1, 16)  OutScaling=2^0
      InputValues=|
      | [0
      |     0.0510
      |     0.1530
      |     0.3080
      |     0.4800
      |     0.6630
      |     0.9110
      |     1.0570
      |     1.2210
      |     1.3740]
      Table=|
      | [0.0500
      |     0.1000
      |     0.2000
      |     0.3000
      |     0.4000
      |     0.5000
      |     0.6000
      |     0.7000
      |     0.8000
      |     0.9000]
  if == 0 : simulink/Logic and Bit Operations/Compare To Zero  SystemSampleTime=-1  relop===  LogicOutDataTypeMode=uint8
  u_1 : Outport
  wires:
  Multiport Switch/1 -> u_1/1
  Gain1/1 -> Sum/3
  Gain/1 -> Sum/2
  Sum/1 -> Multiport Switch/1
  If > 0/1 -> Gain1/1
  if == 0/1 -> Gain/1
  If < 0/1 -> Sum/1
  f_1/1 -> f_1 < 0/1, f_1 > 0/1, Dead Zone/1
  f_1 < 0/1 -> Multiport Switch/2
  f_1 = 0/1 -> Multiport Switch/3
  f_1 > 0/1 -> Multiport Switch/4
  Dead Zone/1 -> If < 0/1, if == 0/1, If > 0/1

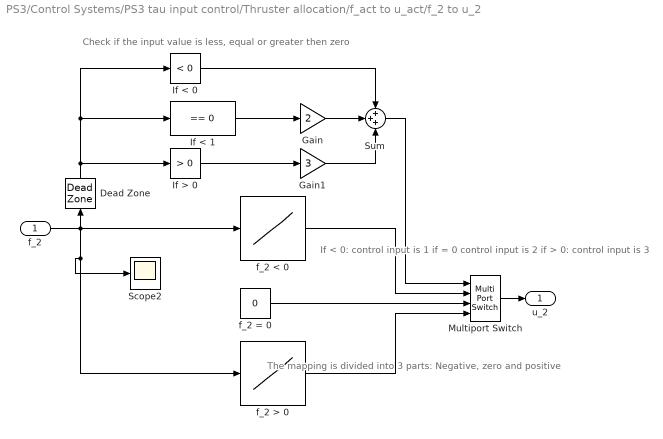
== system PS3/Control Systems/PS3 tau input control/Thruster allocation/f_act to u_act/f_2 to u_2 ==
  note: If < 0: control input is 1
      | if = 0 control input is 2
      | if > 0: control input is 3
  note: Check if the input value is less, equal or greater then zero
  note: The mapping is divided into 3 parts:
      | Negative, zero and positive
  f_2 : Inport
  Dead Zone : DeadZone  LowerValue=-0.001  UpperValue=0.001  SaturateOnIntegerOverflow=on
  Gain : Gain  Gain=2  ParameterDataType=fixdt(1, 16)  ParameterScaling=2^0  OutDataType=fixdt(1, 16)  OutScaling=2^0
  Gain1 : Gain  Gain=3  ParameterDataType=fixdt(1, 16)  ParameterScaling=2^0  OutDataType=fixdt(1, 16)  OutScaling=2^0
  If < 0 : simulink/Logic and Bit Operations/Compare To Constant  SystemSampleTime=-1  relop=<  const=0  LogicOutDataTypeMode=uint8
  If < 1 : simulink/Logic and Bit Operations/Compare To Constant  SystemSampleTime=-1  relop===  const=0  LogicOutDataTypeMode=uint8
  If > 0 : simulink/Logic and Bit Operations/Compare To Constant  SystemSampleTime=-1  relop=>  const=0  LogicOutDataTypeMode=uint8
  Multiport Switch : MultiPortSwitch  OutDataType=fixdt(1, 16)  OutScaling=2^0
  Scope2 : Scope
      settings: SaveName=ScopeData7
  Sum : Sum  Inputs=+++  OutDataType=fixdt(1, 16)  OutScaling=2^0
  f_2 < 0 : Lookup  InputValues=|  Table=|  LookUpMeth=Interpolation-Use End Values  OutDataType=fixdt(1, 16)  OutScaling=2^0
      InputValues=|
      | [-0.766
      | -0.649
      | -0.522
      | -0.411
      | -0.323
      | -0.246
      | -0.156
      | -0.075
      | -0.018
      | -0.006
      | 0]
      Table=|
      | [-1.0000
      |    -0.9000
      |    -0.8000
      |    -0.7000
      |    -0.6000
      |    -0.5000
      |    -0.4000
      |    -0.3000
      |    -0.2000
      |    -0.1000
      |    -0.0466]
  f_2 = 0 : Constant  Value=0  OutDataType=fixdt(1, 16)  OutScaling=2^0
  f_2 > 0 : Lookup  InputValues=|  Table=|  LookUpMeth=Interpolation-Use End Values  OutDataType=fixdt(1, 16)  OutScaling=2^0
      InputValues=|
      | [0.000
      | 0.052
      | 0.207
      | 0.331
      | 0.509
      | 0.689
      | 0.829
      | 0.961
      | 1.079
      | 1.120
      | ]
      Table=|
      | [0.1665
      |     0.2000
      |     0.3000
      |     0.4000
      |     0.5000
      |     0.6000
      |     0.7000
      |     0.8000
      |     0.9000
      |     1.0000]
  u_2 : Outport
  wires:
  f_2 > 0/1 -> Multiport Switch/4
  f_2 = 0/1 -> Multiport Switch/3
  f_2 < 0/1 -> Multiport Switch/2
  f_2/1 -> f_2 < 0/1, f_2 > 0/1, Scope2/1, Dead Zone/1
  If < 0/1 -> Sum/1
  If < 1/1 -> Gain/1
  If > 0/1 -> Gain1/1
  Sum/1 -> Multiport Switch/1
  Gain/1 -> Sum/2
  Gain1/1 -> Sum/3
  Multiport Switch/1 -> u_2/1
  Dead Zone/1 -> If > 0/1, If < 0/1, If < 1/1

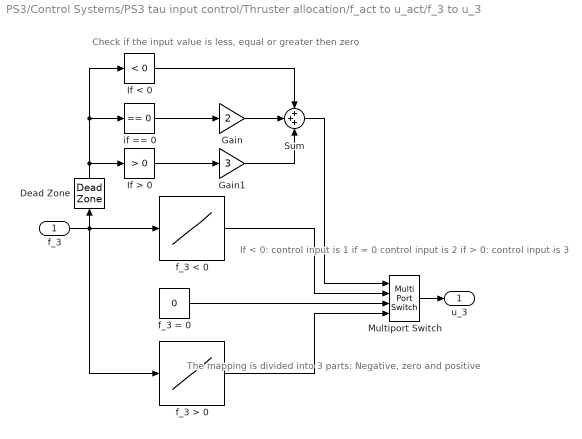
== system PS3/Control Systems/PS3 tau input control/Thruster allocation/f_act to u_act/f_3 to u_3 ==
  note: If < 0: control input is 1
      | if = 0 control input is 2
      | if > 0: control input is 3
  note: Check if the input value is less, equal or greater then zero
  note: The mapping is divided into 3 parts:
      | Negative, zero and positive
  f_3 : Inport
  Dead Zone : DeadZone  LowerValue=-0.001  UpperValue=0.001  SaturateOnIntegerOverflow=on
  Gain : Gain  Gain=2  ParameterDataType=fixdt(1, 16)  ParameterScaling=2^0  OutDataType=fixdt(1, 16)  OutScaling=2^0
  Gain1 : Gain  Gain=3  ParameterDataType=fixdt(1, 16)  ParameterScaling=2^0  OutDataType=fixdt(1, 16)  OutScaling=2^0
  If < 0 : simulink/Logic and Bit Operations/Compare To Constant  SystemSampleTime=-1  relop=<  const=0  LogicOutDataTypeMode=uint8
  If > 0 : simulink/Logic and Bit Operations/Compare To Constant  SystemSampleTime=-1  relop=>  const=0  LogicOutDataTypeMode=uint8
  Multiport Switch : MultiPortSwitch  OutDataType=fixdt(1, 16)  OutScaling=2^0
  Sum : Sum  Inputs=+++  OutDataType=fixdt(1, 16)  OutScaling=2^0
  f_3 < 0 : Lookup  InputValues=|  Table=|  LookUpMeth=Interpolation-Use End Values  OutDataType=fixdt(1, 16)  OutScaling=2^0
      InputValues=|
      | [-1.291
      | -1.088
      | -0.885
      | -0.618
      | -0.403
      | -0.211
      | -0.034
      | 0.000]
      Table=|
      | [-0.9000
      |    -0.8000
      |    -0.7000
      |    -0.6000
      |    -0.5000
      |    -0.4000
      |    -0.3000
      |    -0.2809]
  f_3 = 0 : Constant  Value=0  OutDataType=fixdt(1, 16)  OutScaling=2^0
  f_3 > 0 : Lookup  InputValues=|  Table=|  LookUpMeth=Interpolation-Use End Values  OutDataType=fixdt(1, 16)  OutScaling=2^0
      InputValues=|
      | [0.000
      | 0.014
      | 0.040
      | 0.147
      | 0.302
      | 0.494
      | 0.680
      | 0.968
      | 1.111
      | 1.289
      | 1.339]
      Table=|
      | [0.0452
      |     0.1000
      |     0.2000
      |     0.3000
      |     0.4000
      |     0.5000
      |     0.6000
      |     0.7000
      |     0.8000
      |     0.9000
      |     1.0000
      | ]
  if == 0 : simulink/Logic and Bit Operations/Compare To Zero  SystemSampleTime=-1  relop===  LogicOutDataTypeMode=uint8
  u_3 : Outport
  wires:
  Multiport Switch/1 -> u_3/1
  Gain1/1 -> Sum/3
  Gain/1 -> Sum/2
  Sum/1 -> Multiport Switch/1
  If > 0/1 -> Gain1/1
  if == 0/1 -> Gain/1
  If < 0/1 -> Sum/1
  f_3/1 -> f_3 < 0/1, f_3 > 0/1, Dead Zone/1
  f_3 < 0/1 -> Multiport Switch/2
  f_3 = 0/1 -> Multiport Switch/3
  f_3 > 0/1 -> Multiport Switch/4
  Dead Zone/1 -> If < 0/1, if == 0/1, If > 0/1

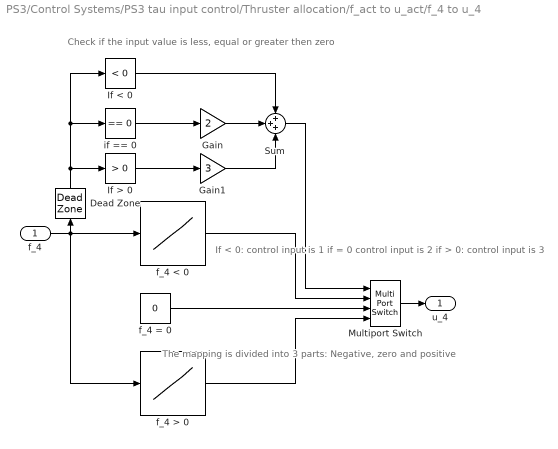
== system PS3/Control Systems/PS3 tau input control/Thruster allocation/f_act to u_act/f_4 to u_4 ==
  note: If < 0: control input is 1
      | if = 0 control input is 2
      | if > 0: control input is 3
  note: Check if the input value is less, equal or greater then zero
  note: The mapping is divided into 3 parts:
      | Negative, zero and positive
  f_4 : Inport
  Dead Zone : DeadZone  LowerValue=-0.001  UpperValue=0.001  SaturateOnIntegerOverflow=on
  Gain : Gain  Gain=2  ParameterDataType=fixdt(1, 16)  ParameterScaling=2^0  OutDataType=fixdt(1, 16)  OutScaling=2^0
  Gain1 : Gain  Gain=3  ParameterDataType=fixdt(1, 16)  ParameterScaling=2^0  OutDataType=fixdt(1, 16)  OutScaling=2^0
  If < 0 : simulink/Logic and Bit Operations/Compare To Constant  SystemSampleTime=-1  relop=<  const=0  LogicOutDataTypeMode=uint8
  If > 0 : simulink/Logic and Bit Operations/Compare To Constant  SystemSampleTime=-1  relop=>  const=0  LogicOutDataTypeMode=uint8
  Multiport Switch : MultiPortSwitch  OutDataType=fixdt(1, 16)  OutScaling=2^0
  Sum : Sum  Inputs=+++  OutDataType=fixdt(1, 16)  OutScaling=2^0
  f_4 < 0 : Lookup  InputValues=|  Table=|  LookUpMeth=Interpolation-Use End Values  OutDataType=fixdt(1, 16)  OutScaling=2^0
      InputValues=|
      | [-1.249
      | -1.225
      | -1.094
      | -0.896
      | -0.696
      | -0.502
      | -0.314
      | -0.169
      | -0.042
      | 0.000]
      Table=|
      | [-0.9000
      |    -0.8000
      |    -0.7000
      |    -0.6000
      |    -0.5000
      |    -0.4000
      |    -0.3000
      |    -0.2000
      |    -0.1000
      |    -0.0674]
  f_4 = 0 : Constant  Value=0  OutDataType=fixdt(1, 16)  OutScaling=2^0
  f_4 > 0 : Lookup  InputValues=|  Table=|  LookUpMeth=Interpolation-Use End Values  OutDataType=fixdt(1, 16)  OutScaling=2^0
      InputValues=|
      | [0.000
      | 0.063
      | 0.107
      | 0.274
      | 0.441
      | 0.599
      | 0.731]
      Table=|
      | [0.3588
      |     0.5000
      |     0.6000
      |     0.7000
      |     0.8000
      |     0.9000
      |     1.0000]
  if == 0 : simulink/Logic and Bit Operations/Compare To Zero  SystemSampleTime=-1  relop===  LogicOutDataTypeMode=uint8
  u_4 : Outport
  wires:
  f_4 > 0/1 -> Multiport Switch/4
  f_4 = 0/1 -> Multiport Switch/3
  f_4 < 0/1 -> Multiport Switch/2
  f_4/1 -> f_4 > 0/1, f_4 < 0/1, Dead Zone/1
  If < 0/1 -> Sum/1
  if == 0/1 -> Gain/1
  If > 0/1 -> Gain1/1
  Sum/1 -> Multiport Switch/1
  Gain/1 -> Sum/2
  Gain1/1 -> Sum/3
  Multiport Switch/1 -> u_4/1
  Dead Zone/1 -> If > 0/1, if == 0/1, If < 0/1

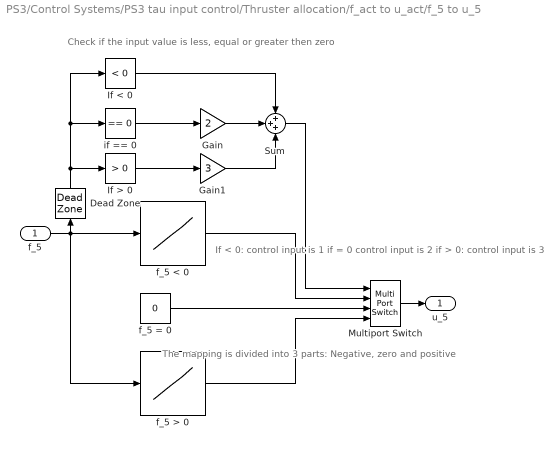
== system PS3/Control Systems/PS3 tau input control/Thruster allocation/f_act to u_act/f_5 to u_5 ==
  note: The mapping is divided into 3 parts:
      | Negative, zero and positive
  note: Check if the input value is less, equal or greater then zero
  note: If < 0: control input is 1
      | if = 0 control input is 2
      | if > 0: control input is 3
  f_5 : Inport
  Dead Zone : DeadZone  LowerValue=-0.001  UpperValue=0.001  SaturateOnIntegerOverflow=on
  Gain : Gain  Gain=2  ParameterDataType=fixdt(1, 16)  ParameterScaling=2^0  OutDataType=fixdt(1, 16)  OutScaling=2^0
  Gain1 : Gain  Gain=3  ParameterDataType=fixdt(1, 16)  ParameterScaling=2^0  OutDataType=fixdt(1, 16)  OutScaling=2^0
  If < 0 : simulink/Logic and Bit Operations/Compare To Constant  SystemSampleTime=-1  relop=<  const=0  LogicOutDataTypeMode=uint8
  If > 0 : simulink/Logic and Bit Operations/Compare To Constant  SystemSampleTime=-1  relop=>  const=0  LogicOutDataTypeMode=uint8
  Multiport Switch : MultiPortSwitch  OutDataType=fixdt(1, 16)  OutScaling=2^0
  Sum : Sum  Inputs=+++  OutDataType=fixdt(1, 16)  OutScaling=2^0
  f_5 < 0 : Lookup  InputValues=|  Table=|  LookUpMeth=Interpolation-Use End Values  OutDataType=fixdt(1, 16)  OutScaling=2^0
      InputValues=|
      | [-1.2630
      |    -1.0309
      |    -0.3808]
      Table=|
      | [-0.3000
      |    -0.2000
      |    -0.1000]
  f_5 = 0 : Constant  Value=0  OutDataType=fixdt(1, 16)  OutScaling=2^0
  f_5 > 0 : Lookup  InputValues=|  Table=|  LookUpMeth=Interpolation-Use End Values  OutDataType=fixdt(1, 16)  OutScaling=2^0
      InputValues=|
      | [0.3480
      |     0.8290
      |     1.0930]
      Table=|
      | [0.1000
      |     0.2000
      |     0.3000]
  if == 0 : simulink/Logic and Bit Operations/Compare To Zero  SystemSampleTime=-1  relop===  LogicOutDataTypeMode=uint8
  u_5 : Outport
  wires:
  Multiport Switch/1 -> u_5/1
  Gain1/1 -> Sum/3
  Gain/1 -> Sum/2
  Sum/1 -> Multiport Switch/1
  If > 0/1 -> Gain1/1
  if == 0/1 -> Gain/1
  If < 0/1 -> Sum/1
  f_5/1 -> f_5 < 0/1, f_5 > 0/1, Dead Zone/1
  f_5 < 0/1 -> Multiport Switch/2
  f_5 = 0/1 -> Multiport Switch/3
  f_5 > 0/1 -> Multiport Switch/4
  Dead Zone/1 -> If < 0/1, if == 0/1, If > 0/1

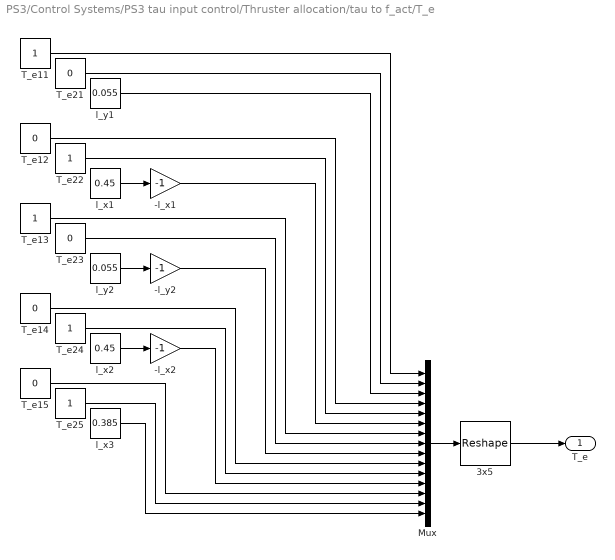
== system PS3/Control Systems/PS3 tau input control/Thruster allocation/tau to f_act/T_e ==
  -l_x1 : Gain  Gain=-1
  -l_x2 : Gain  Gain=-1
  -l_y2 : Gain  Gain=-1
  3x5 : Reshape  OutputDimensionality=Customize  OutputDimensions=[3,5]
  Mux : Mux  Inputs=15
  T_e{11,13,22,24..25} (5 alike) : Constant
  T_e{12,14..15,21,23} (5 alike) : Constant  Value=0
  l_x1 : Constant  Value=0.45
  l_x2 : Constant  Value=0.45
  l_x3 : Constant  Value=0.385
  l_y1 : Constant  Value=0.055
  l_y2 : Constant  Value=0.055
  T_e : Outport
  wires:
  l_x3/1 -> Mux/15
  T_e25/1 -> Mux/14
  T_e15/1 -> Mux/13
  -l_x2/1 -> Mux/12
  -l_y2/1 -> Mux/9
  -l_x1/1 -> Mux/6
  l_x2/1 -> -l_x2/1
  T_e24/1 -> Mux/11
  T_e14/1 -> Mux/10
  l_y2/1 -> -l_y2/1
  T_e23/1 -> Mux/8
  T_e13/1 -> Mux/7
  l_x1/1 -> -l_x1/1
  T_e22/1 -> Mux/5
  T_e12/1 -> Mux/4
  l_y1/1 -> Mux/3
  T_e21/1 -> Mux/2
  T_e11/1 -> Mux/1
  3x5/1 -> T_e/1
  Mux/1 -> 3x5/1
